simulink model "v_a_b_c_to_v_d_q_1_2"  (R2021a)
settings: Solver=VariableStepAuto  StartTime=0.0  StopTime=10.0  RelTol=1e-3
settings Model: Creator=danesh  LastModifiedBy=danesh

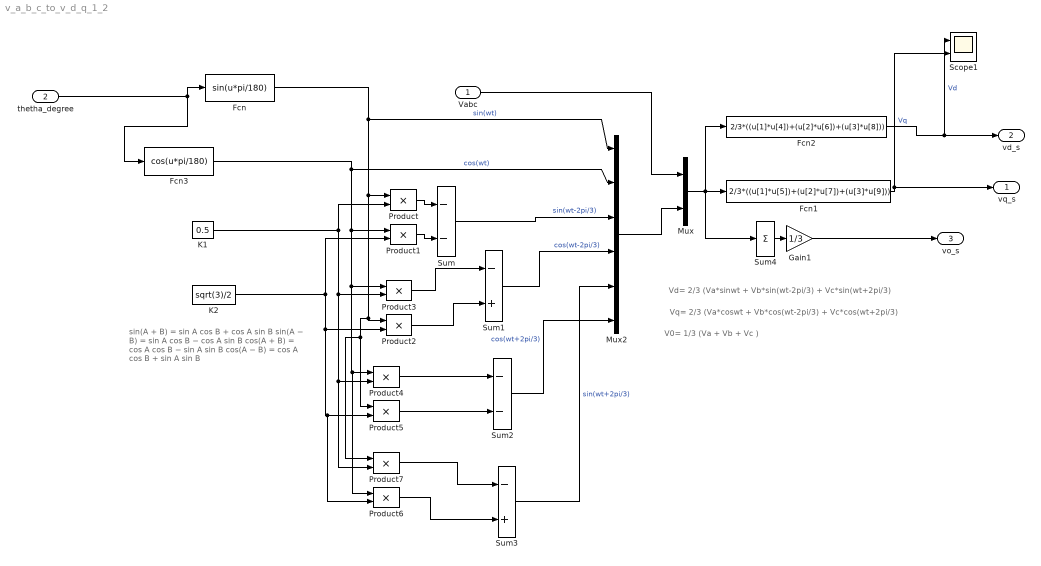
== system v_a_b_c_to_v_d_q_1_2 ==
  note: Vq= 2/3 (Va*coswt + Vb*cos(wt-2pi/3) + Vc*cos(wt+2pi/3)
  note: V0= 1/3 (Va + Vb + Vc )
  note: sin(A + B) = sin A cos B + cos A sin B
      | sin(A − B) = sin A cos B − cos A sin B
      | cos(A + B) = cos A cos B − sin A sin B
      | cos(A − B) = cos A cos B + sin A sin B
  note: Vd= 2/3 (Va*sinwt + Vb*sin(wt-2pi/3) + Vc*sin(wt+2pi/3)
  Vabc : Inport
  thetha_degree : Inport  Port=2
  Fcn : Fcn  Expr=sin(u*pi/180)
  Fcn1 : Fcn  Expr=2/3*((u[1]*u[5])+(u[2]*u[7])+(u[3]*u[9]))
  Fcn2 : Fcn  Expr=2/3*((u[1]*u[4])+(u[2]*u[6])+(u[3]*u[8]))
  Fcn3 : Fcn  Expr=cos(u*pi/180)
  Gain1 : Gain  Gain=1/3  SaturateOnIntegerOverflow=on  OutDataTypeStr=Inherit: Same as input  ParamDataTypeStr=Inherit: Same as input
  K1 : Constant  Value=0.5
  K2 : Constant  Value=sqrt(3)/2
  Mux : Mux  Inputs=2
  Mux2 : Mux  Inputs=6
  Product{,1..7} (8 alike) : Product  InputSameDT=on  SaturateOnIntegerOverflow=on  OutDataTypeStr=Inherit: Same as first input
  Scope1 : Scope  NumInputPorts=2
  Sum : Sum  Inputs=--  InputSameDT=on  SaturateOnIntegerOverflow=on  OutDataTypeStr=Inherit: Same as first input
  Sum1 : Sum  Inputs=-+  InputSameDT=on  SaturateOnIntegerOverflow=on  OutDataTypeStr=Inherit: Same as first input
  Sum2 : Sum  Inputs=--  InputSameDT=on  SaturateOnIntegerOverflow=on  OutDataTypeStr=Inherit: Same as first input
  Sum3 : Sum  Inputs=-+  InputSameDT=on  SaturateOnIntegerOverflow=on  OutDataTypeStr=Inherit: Same as first input
  Sum4 : Sum  Inputs=1  InputSameDT=on  SaturateOnIntegerOverflow=on  OutDataTypeStr=Inherit: Same as first input
  vq_s : Outport  VectorParamsAs1DForOutWhenUnconnected=off
  vd_s : Outport  Port=2  VectorParamsAs1DForOutWhenUnconnected=off
  vo_s : Outport  Port=3  VectorParamsAs1DForOutWhenUnconnected=off
  wires:
  Vabc/1 -> Mux/1
  thetha_degree/1 -> Fcn3/1, Fcn/1
  Sum3/1 -> Mux2/5  "sin(wt+2pi/3)"
  Product3/1 -> Sum1/1
  Product1/1 -> Sum/2
  Product5/1 -> Sum2/2
  Fcn2/1 -> vd_s/1, Scope1/1  "Vd"
  Sum1/1 -> Mux2/4  "cos(wt-2pi/3)"
  Product6/1 -> Sum3/2
  Fcn3/1 -> Product6/1, Product4/1, Product3/1, Product1/1, Mux2/2  "cos(wt)"
  Gain1/1 -> vo_s/1
  Product4/1 -> Sum2/1
  K1/1 -> Product/2, Product7/2, Product4/2, Product3/2
  Sum4/1 -> Gain1/1
  Fcn1/1 -> vq_s/1, Scope1/2  "Vq"
  Sum/1 -> Mux2/3  "sin(wt-2pi/3)"
  K2/1 -> Product1/2, Product6/2, Product5/2, Product2/2
  Sum2/1 -> Mux2/6  "cos(wt+2pi/3)"
  Product7/1 -> Sum3/1
  Mux/1 -> Fcn2/1, Fcn1/1, Sum4/1
  Product2/1 -> Sum1/2
  Mux2/1 -> Mux/2
  Product/1 -> Sum/1
  Fcn/1 -> Product/1, Product7/1, Product5/1, Product2/1, Mux2/1  "sin(wt)"
